simulink model "LLC_Matlab"  (R2016b)
settings: Solver=VariableStepAuto  StartTime=0.0  StopTime=0.04  MaxStep=1e-4  RelTol=1e-3
libraries: powerlib x31
settings Model: SimulationMode=accelerator  Creator=zhengchexiao  LastModifiedBy=zhengchexiao

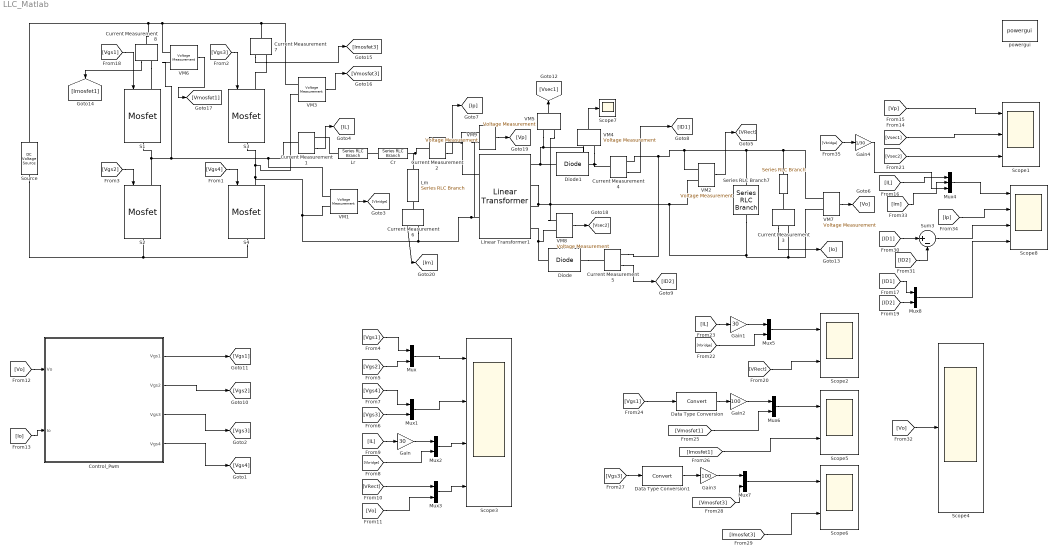
== system LLC_Matlab ==
  " " : powerlib/Elements/Series RLC Branch  LConnTagsString=__new0  RConnTagsString=__new0  BranchType=R  Resistance=(20*20)/2000  Inductance=1e-3  SetiL0=off  InitialCurrent=0  Capacitance=1e-6  Setx0=off  InitialVoltage=0  Measurements=None
  Control_Pwm : Subsystem
  Cr : powerlib/Elements/Series RLC Branch  LConnTagsString=__new0  RConnTagsString=__new0  BranchType=C  Resistance=0.03  Inductance=20e-6  SetiL0=off  InitialCurrent=0  Capacitance=88e-9  Setx0=off  InitialVoltage=0  Measurements=None
  Current Measurement{1..8} (8 alike) : powerlib/Measurements/Current Measurement  Tag=PoWeRsYsTeMmEaSuReMeNt  PhasorSimulation=off  OutputType=Magnitude  PSBequivalent=0
  Data Type Conversion : DataTypeConversion
  Data Type Conversion1 : DataTypeConversion
  Diode : powerlib/Power Electronics/Diode  Ron=0.001  Lon=0  Vf=0.8  IC=0  UseSnubber=off  Rs=500  Cs=250e-9  Measurements=off
  Diode1 : powerlib/Power Electronics/Diode  Ron=0.001  Lon=0  Vf=0.8  IC=0  UseSnubber=off  Rs=500  Cs=250e-9  Measurements=off
  Gain : Gain  Gain=30
  Gain1 : Gain  Gain=30
  Gain2 : Gain  Gain=100
  Gain3 : Gain  Gain=100
  Gain4 : Gain  Gain=1/30
  Linear Transformer1 : powerlib/Elements/Linear Transformer  UNITS=SI  NominalPower=[500e3 1]  winding1=[13 0 0]  winding2=[1 0 0]  ThreeWindings=on  winding3=[1 0 0]  RmLm=[9e6 0]  Measurements=Winding voltages  DataType=on
  Lm : powerlib/Elements/Series RLC Branch  LConnTagsString=__new0  RConnTagsString=__new0  BranchType=L  Resistance=0.03  Inductance=66e-6  SetiL0=off  InitialCurrent=0  Capacitance=1e-6  Setx0=off  InitialVoltage=0  Measurements=None
  Lr : powerlib/Elements/Series RLC Branch  LConnTagsString=__new0  RConnTagsString=__new0  BranchType=L  Resistance=0.03  Inductance=20e-6  SetiL0=off  InitialCurrent=0  Capacitance=1e-6  Setx0=off  InitialVoltage=0  Measurements=None
  Mux{,1..3,5..8} (8 alike) : Mux  Inputs=2
  Mux4 : Mux  Inputs=3
  S{1..4} (4 alike) : powerlib/Power Electronics/Mosfet  Ron=0.001  Lon=0  Rd=0.01  Vfd=0.7  IC=0  Rs=1e2  Cs=0  Measurements=off
  Scope1 : Scope  NumInputPorts=3
  Scope2 : Scope  NumInputPorts=2
  Scope3 : Scope  NumInputPorts=4
  Scope4 : Scope
  Scope5 : Scope  NumInputPorts=2
  Scope6 : Scope  NumInputPorts=2
  Scope7 : Scope
  Scope8 : Scope  NumInputPorts=4
  Series RLC Branch7 : powerlib/Elements/Series RLC Branch  LConnTagsString=__new0  RConnTagsString=__new0  BranchType=C  Resistance=1.0  Inductance=1.0  SetiL0=off  InitialCurrent=0  Capacitance=1000e-6  Setx0=on  InitialVoltage=15  Measurements=None
  Source : powerlib/Electrical Sources/DC Voltage Source  Amplitude=325  Measurements=None
  Sum3 : Sum  Inputs=|+-
  VM{1..9} (9 alike) : powerlib/Measurements/Voltage Measurement  PhasorSimulation=off  OutputType=Complex  PSBequivalent=0
  powergui : powerlib/powergui  Priority=1  SimulationMode=Continuous  SampleTime=10e-9  frequency=60  Iterations=50  frequencyindice=0  Pbase=100e6  ErrMax=1e-4  UnitsV=kV  UnitsW=MW  buscounter=0  FunctionMessages=off  echomessages=off  EnableUseOfTLC=off  CurrentSourceSwitches=off  DisableSnubberDevices=off  DisableRonSwitches=off  DisableVfSwitches=off  DisplayEquations=off  SolverType=Tustin/Backward Euler (TBE)  Interpol=off  ExternalGateDelay=off  methode=off  Ts=100  x0status=blocks  SPID=on  SwTol=0  HookPort=off  RestoreLinks=warning  ResistiveCurrentMeasurement=off  Frange=[0:2:500]  Ylog=off  Xlog=on  ShowGrid=off  save=off  variable=ZData  structure=0  ZoomFFT=off  StartTime=0.0  cycles=1  DisplayStyle=1  fundamental=60  FreqAxis=off  MaxFrequency=1000  frequencyindicesteady=1  RmsSteady=1  display=off
  wires:
  [Vgs1] -> S1/1
  [Vgs4] -> S4/1
  [Vgs3] -> S3/1
  [Vgs2] -> S2/1
  VM7/1 -> [Vo]
  [Vgs1] -> Mux/1
  [Vgs2] -> Mux/2
  Mux/1 -> Scope3/1
  Mux1/1 -> Scope3/2
  VM1/1 -> [Vbridge]
  Current Measurement1/1 -> [IL]
  [IL] -> Gain/1
  Gain/1 -> Mux2/1
  [Vbridge] -> Mux2/2
  Mux2/1 -> Scope3/3
  VM2/1 -> [VRect]
  [VRect] -> Mux3/1
  Mux3/1 -> Scope3/4
  [Vo] -> Mux3/2
  [Vgs4] -> Mux1/1
  [Vgs3] -> Mux1/2
  Control_Pwm/1(Vgs1) -> [Vgs1]
  Control_Pwm/2(Vgs2) -> [Vgs2]
  Control_Pwm/3(Vgs3) -> [Vgs3]
  Control_Pwm/4(Vgs4) -> [Vgs4]
  [Vo] -> Control_Pwm/1(Vo)
  Current Measurement4/1 -> [ID1]
  Current Measurement5/1 -> [ID2]
  [Io] -> Control_Pwm/2(Io)
  Current Measurement3/1 -> [Io]
  Mux5/1 -> Scope2/1
  [Vbridge] -> Mux5/2
  Gain1/1 -> Mux5/1
  [IL] -> Gain1/1
  [VRect] -> Scope2/2
  Gain2/1 -> Mux6/1
  [Vgs1] -> Data Type Conversion/1
  [Vmosfet1] -> Mux6/2
  Mux6/1 -> Scope5/1
  [Imosfet1] -> Scope5/2
  [Imosfet3] -> Scope6/2
  Mux7/1 -> Scope6/1
  [Vmosfet3] -> Mux7/2
  [Vgs3] -> Data Type Conversion1/1
  Gain3/1 -> Mux7/1
  VM3/1 -> [Vmosfet3]
  Current Measurement7/1 -> [Imosfet3]
  Data Type Conversion/1 -> Gain2/1
  Data Type Conversion1/1 -> Gain3/1
  Current Measurement8/1 -> [Imosfet1]
  VM6/1 -> [Vmosfet1]
  [ID2] -> Mux8/2
  [ID1] -> Mux8/1
  [ID2] -> Sum3/2
  [ID1] -> Sum3/1
  VM5/1 -> [Vsec1]
  VM9/1 -> [Vp]
  [Vsec1] -> Scope1/2
  [Vsec2] -> Scope1/3
  [Vp] -> Scope1/1
  VM8/1 -> [Vsec2]
  [Vo] -> Scope4/1
  VM4/1 -> Scope7/1
  Current Measurement2/1 -> [Ip]
  Current Measurement6/1 -> [Im]
  [IL] -> Mux4/1
  [Im] -> Mux4/2
  Mux4/1 -> Scope8/1
  Sum3/1 -> Scope8/3
  Mux8/1 -> Scope8/4
  [Ip] -> Scope8/2
  [Vbridge] -> Gain4/1
  Gain4/1 -> Mux4/3
  connections:
  VM1/LConn1 -- Current Measurement1/LConn1 -- S2/LConn1 -- S1/RConn1 -- VM6/LConn2
  S3/RConn1 -- VM3/LConn2 -- Current Measurement6/RConn1 -- VM9/LConn2 -- Linear Transformer1/LConn2 -- VM1/LConn2 -- S4/LConn1
  Source/RConn1 -- Current Measurement7/LConn1 -- VM3/LConn1 -- VM6/LConn1 -- Current Measurement8/LConn1
  Source/LConn1 -- S4/RConn1 -- S2/RConn1
  Diode/RConn1 -- Current Measurement5/LConn1
  Diode1/RConn1 -- Current Measurement4/LConn1 -- VM4/LConn2
  Diode/LConn1 -- VM8/LConn2 -- Linear Transformer1/RConn4
  Diode1/LConn1 -- VM4/LConn1 -- VM5/LConn1 -- Linear Transformer1/RConn1
  Current Measurement5/RConn1 -- Series RLC Branch7/LConn1 -- VM7/LConn1 -- " "/LConn1 -- VM2/LConn1 -- Current Measurement4/RConn1
  Series RLC Branch7/RConn1 -- Current Measurement3/RConn1 -- VM7/LConn2 -- VM2/LConn2 -- VM5/LConn2 -- VM8/LConn1 -- Linear Transformer1/RConn3 -- Linear Transformer1/RConn2
  Cr/RConn1 -- Lm/LConn1 -- Current Measurement2/LConn1
  Current Measurement3/LConn1 -- " "/RConn1
  Lr/LConn1 -- Current Measurement1/RConn1
  Current Measurement7/RConn1 -- S3/LConn1
  Current Measurement8/RConn1 -- S1/LConn1
  Cr/LConn1 -- Lr/RConn1
  Current Measurement2/RConn1 -- VM9/LConn1 -- Linear Transformer1/LConn1
  Lm/RConn1 -- Current Measurement6/LConn1

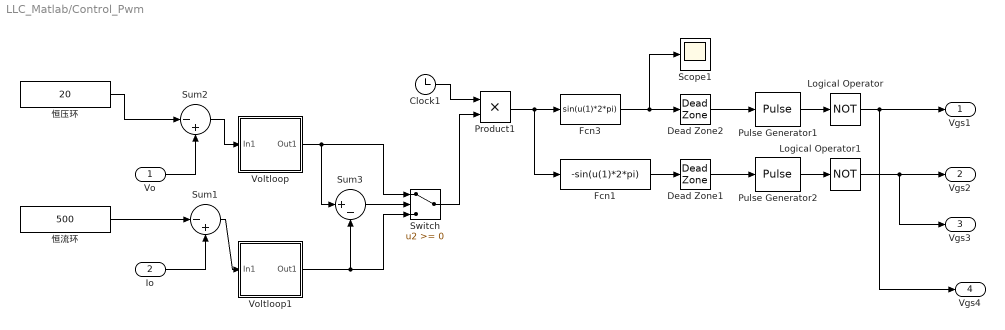
== system LLC_Matlab/Control_Pwm ==
  Vo : Inport
  Io : Inport  Port=2
  Clock1 : Clock
  Dead Zone1 : DeadZone  LowerValue=-0.01  UpperValue=0.01  SaturateOnIntegerOverflow=on
  Dead Zone2 : DeadZone  LowerValue=-0.01  UpperValue=0.01  SaturateOnIntegerOverflow=on
  Fcn1 : Fcn  Expr=-sin(u(1)*2*pi)
  Fcn3 : Fcn  Expr=sin(u(1)*2*pi)
  Logical Operator : Logic  Operator=NOT  AllPortsSameDT=off  OutDataTypeStr=boolean
  Logical Operator1 : Logic  Operator=NOT  AllPortsSameDT=off  OutDataTypeStr=boolean
  Product1 : Product  RndMeth=Zero
  Pulse Generator1 : DiscretePulseGenerator  PulseType=Time based  TimeSource=Use external signal  PulseWidth=50
  Pulse Generator2 : DiscretePulseGenerator  PulseType=Time based  TimeSource=Use external signal  PulseWidth=50
  Scope1 : Scope
  Sum1 : Sum  Inputs=|-+
  Sum2 : Sum  Inputs=|-+
  Sum3 : Sum  Inputs=|+-
  Switch : Switch
  Voltloop : Subsystem
  Voltloop1 : Subsystem
  恒压环 : Constant  Value=20
  恒流环 : Constant  Value=500
  Vgs1 : Outport
  Vgs2 : Outport  Port=2
  Vgs3 : Outport  Port=3
  Vgs4 : Outport  Port=4
  wires:
  Fcn3/1 -> Scope1/1, Dead Zone2/1
  Clock1/1 -> Product1/1
  Fcn1/1 -> Dead Zone1/1
  Dead Zone1/1 -> Pulse Generator2/1
  Product1/1 -> Fcn1/1, Fcn3/1
  Pulse Generator2/1 -> Logical Operator1/1
  Pulse Generator1/1 -> Logical Operator/1
  Dead Zone2/1 -> Pulse Generator1/1
  Sum2/1 -> Voltloop/1(In1)
  Logical Operator1/1 -> Vgs3/1, Vgs2/1
  Logical Operator/1 -> Vgs4/1, Vgs1/1
  恒压环/1 -> Sum2/1
  Vo/1 -> Sum2/2
  恒流环/1 -> Sum1/1
  Io/1 -> Sum1/2
  Sum1/1 -> Voltloop1/1(In1)
  Voltloop/1(Out1) -> Sum3/1, Switch/1
  Voltloop1/1(Out1) -> Sum3/2, Switch/3
  Sum3/1 -> Switch/2
  Switch/1 -> Product1/2

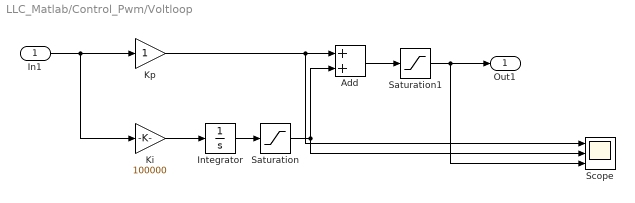
== system LLC_Matlab/Control_Pwm/Voltloop ==
  In1 : Inport
  Add : Sum
  Integrator : Integrator  InitialCondition=152e3
  Ki : Gain  Gain=100000
  Kp : Gain
  Saturation : Saturate  UpperLimit=200e3  LowerLimit=80e3
  Saturation1 : Saturate  UpperLimit=200e3  LowerLimit=80e3
  Scope : Scope  NumInputPorts=3
  Out1 : Outport
  wires:
  Saturation1/1 -> Out1/1, Scope/3
  Add/1 -> Saturation1/1
  Saturation/1 -> Add/2, Scope/2
  Kp/1 -> Add/1, Scope/1
  In1/1 -> Ki/1, Kp/1
  Integrator/1 -> Saturation/1
  Ki/1 -> Integrator/1

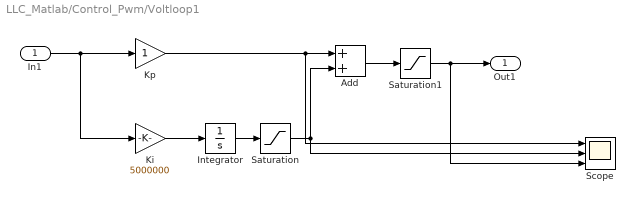
== system LLC_Matlab/Control_Pwm/Voltloop1 ==
  In1 : Inport
  Add : Sum
  Integrator : Integrator  InitialCondition=150e3
  Ki : Gain  Gain=5000000
  Kp : Gain
  Saturation : Saturate  UpperLimit=200e3  LowerLimit=80e3
  Saturation1 : Saturate  UpperLimit=200e3  LowerLimit=80e3
  Scope : Scope  NumInputPorts=3
  Out1 : Outport
  wires:
  Ki/1 -> Integrator/1
  Integrator/1 -> Saturation/1
  In1/1 -> Kp/1, Ki/1
  Kp/1 -> Scope/1, Add/1
  Saturation/1 -> Scope/2, Add/2
  Add/1 -> Saturation1/1
  Saturation1/1 -> Scope/3, Out1/1
